simulink model "DCMoter"  (R2019b)
settings: Solver=VariableStepAuto  StartTime=0.0  StopTime=10.0  RelTol=1e-3
values from neighbouring files (symbols this model uses):
  b = 1e-6    (= 1e-06)    [DCMoterPara.m]
  Jm = 5.6/1000/10000    (= 5.6e-07)    [DCMoterPara.m]
  Ke = 0.6*10^(-3)/(2*pi/60)    (= 0.00572957795131)    [DCMoterPara.m]
  Kt = 5.77*10^(-3)    (= 0.00577)    [DCMoterPara.m]
  La = 13.5*10^(-6)    (= 1.35e-05)    [DCMoterPara.m]
  Ra = 0.4    [DCMoterPara.m]
undefined symbols (not defined in the file or in its folder): sigbuilder_block
settings Model: Creator=23731  LastModifiedBy=23731

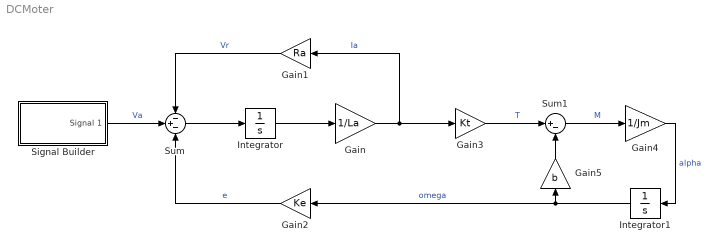
== system DCMoter ==
  Gain : Gain  Gain=1/La
  Gain1 : Gain  Gain=Ra
  Gain2 : Gain  Gain=Ke
  Gain3 : Gain  Gain=Kt
  Gain4 : Gain  Gain=1/Jm
  Gain5 : Gain  Gain=b
  Integrator : Integrator
  Integrator1 : Integrator
  Signal Builder : Subsystem  Tag=STV Subsys  LoadFcn=sigbuilder_block('load');  StartFcn=sigbuilder_block('start');  StopFcn=sigbuilder_block('stop');  ClipboardFcn=sigbuilder_block('clipboard');  mask(Sigbuilder block){tuvar=[0:10]}
      mask help: Simulink:masks:SigbuilderBlock_MD
      mask init:
      | if ~strcmp(get_param(bdroot(gcbh),'SimulationStatus'),'stopped') tuvar = sigbuilder_block('maskInit'); end
      settings: CopyFcn=sigbuilder_block('copy');  DeleteFcn=sigbuilder_block('delete');  ModelCloseFcn=sigbuilder_block('modelClose');  PreSaveFcn=sigbuilder_block('preSave');  PauseFcn=sigbuilder_block('pause');  ContinueFcn=sigbuilder_block('continue');  NameChangeFcn=sigbuilder_block('namechange');  OpenFcn=sigbuilder_block('open',[437.6 199.2 550.4 400 ]);  CloseFcn=sigbuilder_block('close');
      mask Display: plot(0, 0, 100, 100,[2, 2, 32, 32, 2], [68, 8, 8, 68, 68],[32, 2], [38, 38], [32, 19, 2],[53, 60, 44], [32, 17, 17, 2],[16, 16, 31, 31]);txt = getActiveGroup(gcbh);text(2, 100, txt,'verticalAlignment', 'top');
  Sum : Sum  Inputs=-+-
  Sum1 : Sum  Inputs=|+-
  wires:
  Sum/1 -> Integrator/1
  Integrator/1 -> Gain/1
  Signal Builder/1(Signal 1) -> Sum/2  "Va"
  Gain/1 -> Gain3/1, Gain1/1  "Ia"
  Gain1/1 -> Sum/1  "Vr"
  Gain2/1 -> Sum/3  "e"
  Gain3/1 -> Sum1/1  "T"
  Sum1/1 -> Gain4/1  "M"
  Gain4/1 -> Integrator1/1  "alpha"
  Gain5/1 -> Sum1/2
  Integrator1/1 -> Gain5/1, Gain2/1  "omega"

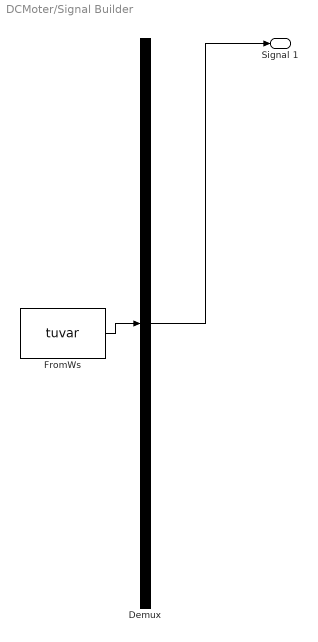
== system DCMoter/Signal Builder ==
  Demux : Demux  Tag=STV Demux  Outputs=1
  FromWs : FromWorkspace  Tag=STV FromWs  VariableName=tuvar  SampleTime=0
      SigBuilderData=|
      | common.afterFinalStr = 'Extrapolate'
      | common.sampleTime = 0
      | dataSet.timeRange = [0 10]
      | dataSet.name = 'Group 1'
      | sbobj.Groups.Name = 'Group 1'
      | sbobj.Groups.Signals.Name = 'Signal 1'
      | sbobj.Groups.Signals.XData = [0 4 4 6 6 10]
      | sbobj.Groups.Signals.YData = [0 0 1 1 0 0]
  Signal 1 : Outport  Tag=STV Outport
  wires:
  Demux/1 -> Signal 1/1
  FromWs/1 -> Demux/1
